simulink library "csc_eap_evaluate_ap_lib"  (R2014b)
settings: Solver=ode45  StartTime=0.0  StopTime=10.0  RelTol=1e-3
libraries: util_common_lib x4, simulink x2, util_event_lib x2, util_info_lib x1, csu_rpn_ap_rpn_evaluation_lib x1
settings Model: Creator=escrane  LastModifiedBy=mstewart

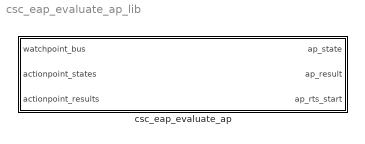
== system csc_eap_evaluate_ap_lib ==
  csc_eap_evaluate_ap : Subsystem  mask{ap_id=1, ap_start_rts_id=5, ap_max_fail_before_rts=1, ap_wp_equation=1 2 NOT AND, ap_default_state=DISABLED, ap_event_type=CRITICAL, ap_event_id=20, ap_event_text='AP failed, starting RTS 5'}
      mask prompts: ap_id "ID number (1-255) of Action Point"; ap_start_rts_id "ID number of RTS to start on AP fail"; ap_max_fail_before_rts "Number of consecutive failures before RTS call"; ap_wp_equation "Watchpoint Equation Vector (numeric postfix notation)"; ap_default_state "Default State of AP"; ap_event_type "Event Type"; ap_event_id "Event ID"; ap_event_text "Event Text (no format specifiers allowed, use %% for a percent sign)"
      mask init:
      | csc_eap_evaluate_ap_callback(gcb, ap_wp_equation, ap_event_type);
      mask TypeOptions ap_default_state: DISABLED | PASSIVE | ACTIVE
      mask TypeOptions ap_event_type: DEBUG | INFORMATION | ERROR | CRITICAL
      mask Display:
      | disp(['{\bfAP #' int2str(ap_id) '}'], 'texmode', 'on');
      | disp(['{\newline\bf= ' ap_wp_equation '}'], 'texmode', 'on');

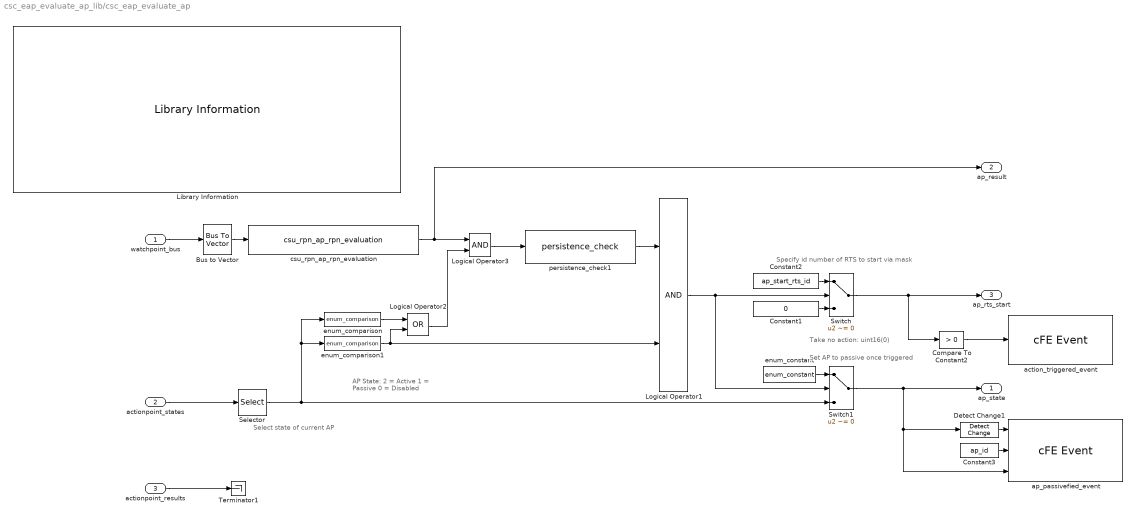
== system csc_eap_evaluate_ap_lib/csc_eap_evaluate_ap ==
  note: AP State:
      | 2 =  Active
      | 1 = Passive
      | 0 = Disabled
  note: Set AP to passive once triggered
  note: Take no action: uint16(0)
  note: Specify id number of RTS to start via mask
  note: Select state of current AP
  watchpoint_bus : Inport
  actionpoint_states : Inport  Port=2
  actionpoint_results : Inport  Port=3
  Bus to Vector : BusToVector
  Compare To Constant2 : simulink/Logic and Bit Operations/Compare To Constant  relop=>  const=0  OutDataTypeStr=boolean
  Constant1 : Constant  Value=0  OutDataTypeStr=uint16
  Constant2 : Constant  Value=ap_start_rts_id  OutDataTypeStr=uint16
  Constant3 : Constant  Value=ap_id  OutDataTypeStr=uint8
  Detect Change1 : simulink/Logic and Bit Operations/Detect Change  vinit=ap_default_state-1  InputProcessing=Inherited  OutDataTypeStr=boolean
  Library Information : util_info_lib/Library Information  owner='NONE'
  Logical Operator1 : Logic  AllPortsSameDT=off  OutDataTypeStr=boolean
  Logical Operator2 : Logic  Operator=OR  AllPortsSameDT=off  OutDataTypeStr=boolean
  Logical Operator3 : Logic  AllPortsSameDT=off  OutDataTypeStr=boolean
  Selector : Selector  Indices=ap_id
  Switch : Switch  Criteria=u2 ~= 0
  Switch1 : Switch  Criteria=u2 ~= 0
  Terminator1 : Terminator
  action_triggered_event : util_event_lib/cFE Event  event_message=ap_event_text  event_id=ap_event_id  event_severity=CRITICAL  event_use_enums=off  event_enum_types={}
  ap_passivefied_event : util_event_lib/cFE Event  event_message='AP %u set to %s'  event_id=21  event_severity=INFORMATION  event_use_enums=on  event_enum_types={'', 'enum_ap_state'}
  csu_rpn_ap_rpn_evaluation : csu_rpn_ap_rpn_evaluation_lib/csu_rpn_ap_rpn_evaluation  rpn_equation=1 2 NOT AND
  enum_comparison : util_common_lib/enum_comparison  comparison_type===
  enum_comparison1 : util_common_lib/enum_comparison  comparison_type===
  enum_constant : util_common_lib/enum_constant
  persistence_check1 : util_common_lib/persistence_check  persistence_limit=ap_max_fail_before_rts
  ap_state : Outport
  ap_result : Outport  Port=2
  ap_rts_start : Outport  Port=3
  wires:
  Compare To Constant2/1 -> action_triggered_event/1
  watchpoint_bus/1 -> Bus to Vector/1
  csu_rpn_ap_rpn_evaluation/1 -> ap_result/1, Logical Operator3/1
  Constant1/1 -> Switch/3
  Constant2/1 -> Switch/1
  Switch/1 -> ap_rts_start/1, Compare To Constant2/1
  enum_constant/1 -> Switch1/1
  Logical Operator1/1 -> Switch/2, Switch1/2
  Switch1/1 -> Detect Change1/1, ap_passivefied_event/3, ap_state/1
  actionpoint_states/1 -> Selector/1
  persistence_check1/1 -> Logical Operator1/1
  enum_comparison/1 -> Logical Operator2/1
  enum_comparison1/1 -> Logical Operator1/2, Logical Operator2/2
  Logical Operator3/1 -> persistence_check1/1
  Logical Operator2/1 -> Logical Operator3/2
  actionpoint_results/1 -> Terminator1/1
  Bus to Vector/1 -> csu_rpn_ap_rpn_evaluation/1
  Selector/1 -> Switch1/3, enum_comparison1/1, enum_comparison/1
  Detect Change1/1 -> ap_passivefied_event/1
  Constant3/1 -> ap_passivefied_event/2
